simulink model "ssc_opamp_inverting"  (R2016a)
settings: Solver=ode15s  StartTime=0.0  StopTime=0.002  MaxStep=0.00002  RelTol=1e-3  AbsTol=1e-3
libraries: fl_lib x9, nesl_utility x3
CloseFcn:
  | try,close(h1_ssc_opamp_inverting),end
  | clear simlog_ssc_opamp_inverting
Description:
  | Op-Amp Circuit - Inverting Amplifier
  | 
  | Copyright 2008-2016 The MathWorks, Inc.
settings Model: Creator=MathWorks  LastModifiedBy=hakan
settings DataIOCC: LimitDataPoints=on  SaveFormat=Array
settings DebuggingCC: SolverPrmCheckMsg=warning  AllowSymbolicDim=off
settings HardwareCC: ProdBitPerPointer=32  ProdLargestAtomicFloat=None  ProdIntDivRoundTo=Undefined  ProdEndianess=Unspecified  ProdWordSize=32  ProdHWDeviceType=32-bit Generic
settings ModelReferenceCC: PropagateSignalLabelsOutOfModel=off
settings ConfigComp: CovModelRefEnable=Off  CovSFcnEnable=off
settings SimscapeCC: SimscapeLogType=all  SimscapeLogSimulationStatistics=on  SimscapeLogName=simlog_ssc_opamp_inverting  SimscapeLogDataHistory=10000

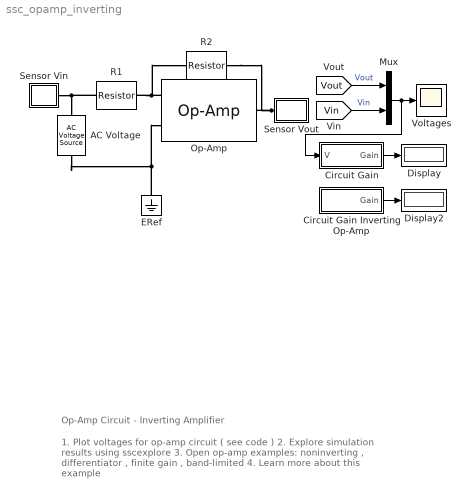
== system ssc_opamp_inverting ==
  note: 1. Plot voltages for op-amp circuit ( see code )
      | 2. Explore simulation results using sscexplore
      | 3. Open op-amp examples:
      | noninverting , differentiator , finite gain , band-limited
      | 4. Learn more about this example
  note: Op-Amp Circuit - Inverting Amplifier
  AC Voltage : fl_lib/Electrical/Electrical Sources/AC Voltage Source  amp=0.1 V  shift=0 deg  frequency=1000 Hz  omega=0 rad/s
  Circuit Gain : Subsystem
  Circuit Gain Inverting Op-Amp : Subsystem
      mask init:
      | set_param([gcb '/R1'],'Value',...
      |     get_param([bdroot '/R1'],'r'));
      | set_param([gcb '/R2'],'Value',...
      |     get_param([bdroot '/R2'],'r'));
      mask Display: disp('-R2/R1')
  Display : Display
  Display2 : Display
  ERef : fl_lib/Electrical/Electrical Elements/Electrical Reference
  Mux : Mux  Inputs=2
  Op-Amp : fl_lib/Electrical/Electrical Elements/Op-Amp  outI_specify=off  outI_priority=High  outI=0 A
  R1 : fl_lib/Electrical/Electrical Elements/Resistor  R=1e3 Ohm  i_specify=off  i_priority=High  i=0 A  v_specify=off  v_priority=High  v=0 V
      settings: AttributesFormatString=%<R> %<R_unit>
  R2 : fl_lib/Electrical/Electrical Elements/Resistor  R=10e3 Ohm  i_specify=off  i_priority=High  i=0 A  v_specify=off  v_priority=High  v=0 V
      settings: AttributesFormatString=%<R> %<R_unit>
  Sensor Vin : Subsystem
      mask Display: disp('Vin')
  Sensor Vout : Subsystem
      mask Display: disp('Vout')
  Voltages : Scope
  wires:
  Mux/1 -> Circuit Gain/1(V), Voltages/1
  [Vout] -> Mux/1  "Vout"
  [Vin] -> Mux/2  "Vin"
  Circuit Gain/1(Gain) -> Display/1
  Circuit Gain Inverting Op-Amp/1(Gain) -> Display2/1
  connections:
  AC Voltage/RConn1 -- ERef/LConn1 -- Op-Amp/LConn1
  R1/LConn1 -- Sensor Vin/LConn1 -- AC Voltage/LConn1
  Op-Amp/LConn2 -- R2/LConn1 -- R1/RConn1
  Op-Amp/RConn1 -- R2/RConn1 -- Sensor Vout/LConn1

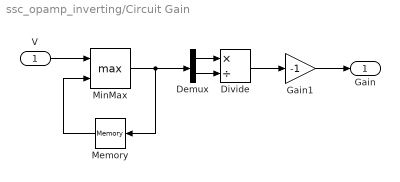
== system ssc_opamp_inverting/Circuit Gain ==
  V : Inport
  Demux : Demux  Outputs=2
  Divide : Product  Inputs=*/
  Gain1 : Gain  Gain=-1
  Memory : Memory  X0=1e-15  InheritSampleTime=on
  MinMax : MinMax  DisableCoverage=on  Function=max  Inputs=2  OutDataTypeStr=Inherit: Inherit via back propagation  ZeroCross=off
      settings: LockScale=on
  Gain : Outport
  wires:
  Gain1/1 -> Gain/1
  Divide/1 -> Gain1/1
  Demux/2 -> Divide/2
  Memory/1 -> MinMax/2
  MinMax/1 -> Demux/1, Memory/1
  Demux/1 -> Divide/1
  V/1 -> MinMax/1

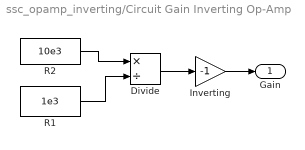
== system ssc_opamp_inverting/Circuit Gain Inverting Op-Amp ==
  Divide : Product  Inputs=*/
  Inverting : Gain  Gain=-1
  R1 : Constant  Value=1e3
  R2 : Constant  Value=10e3
  Gain : Outport
  wires:
  R2/1 -> Divide/1
  R1/1 -> Divide/2
  Inverting/1 -> Gain/1
  Divide/1 -> Inverting/1

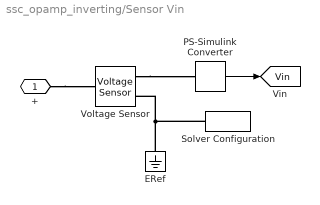
== system ssc_opamp_inverting/Sensor Vin ==
  ERef : fl_lib/Electrical/Electrical Elements/Electrical Reference
  PS-Simulink Converter : nesl_utility/PS-Simulink Converter  PhysicalDomain=network_engine_domain  SubClassName=ps_output  LeftPortType=input  RightPortType=output  PseudoPeriodic=off  Frequencies=[]  Unit=1  AffineConversion=off
  Solver Configuration : nesl_utility/Solver Configuration  PhysicalDomain=network_engine_domain  SubClassName=solver  LeftPortType=input  RightPortType=generic  Accelerate=off  Tones=[]  Harmonics=[]  SimulateNoise=off  Profile=off  UseLocalSampling=off  EnableSwitchedLinearOptims=on  FrequencyDomain=off  UseCCode=off  RelTol=0.001  AbsTol=1e-06  MinStep=1e-09  ToWorkspace=off  RevertToSquareIcSolve=off  NumHomotopyIterations=100  PhasorMode=off  PhasorModeNumHarmonics=1  OverrideAbsTol=off  DoDC=off  ResidualTolerance=1e-9  UseLocalSolver=off  LocalSolverChoice=NE_BACKWARD_EULER_ADVANCER  LocalSolverSampleTime=1e-6  DoFixedCost=off  MaxNonlinIter=3  MaxModeIter=2  LinearAlgebra=Sparse  DelaysMemoryBudget=1024  AutomaticFiltering=on  FilteringTimeConstant=0.001
  Voltage Sensor : fl_lib/Electrical/Electrical Sensors/Voltage Sensor
  + : PMIOPort  Port=1  Side=Left
  tag scope: Vin=global
  wires:
  PS-Simulink Converter/1 -> [Vin]
  connections:
  +/RConn1 -- Voltage Sensor/LConn1
  Voltage Sensor/RConn1 -- PS-Simulink Converter/LConn1
  ERef/LConn1 -- Solver Configuration/RConn1 -- Voltage Sensor/RConn2

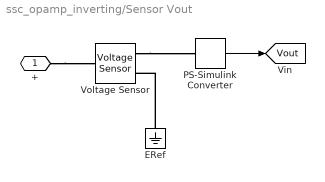
== system ssc_opamp_inverting/Sensor Vout ==
  ERef : fl_lib/Electrical/Electrical Elements/Electrical Reference
  PS-Simulink Converter : nesl_utility/PS-Simulink Converter  PhysicalDomain=network_engine_domain  SubClassName=ps_output  LeftPortType=input  RightPortType=output  PseudoPeriodic=off  Frequencies=[]  Unit=1  AffineConversion=off
  Voltage Sensor : fl_lib/Electrical/Electrical Sensors/Voltage Sensor
  + : PMIOPort  Port=1  Side=Left
  tag scope: Vout=global
  wires:
  PS-Simulink Converter/1 -> [Vout]
  connections:
  ERef/LConn1 -- Voltage Sensor/RConn2
  Voltage Sensor/RConn1 -- PS-Simulink Converter/LConn1
  +/RConn1 -- Voltage Sensor/LConn1
